simulink model "SYSTEM"  (R2026a)
settings: Solver=VariableStepAuto
model workspace (MAT data in the model file):
  CompAir_P : Simulink.ConnectionBus (value not decoded)
  CompAir_S : Simulink.Bus (value not decoded)
  Control_P : Simulink.ConnectionBus (value not decoded)
  Control_S : Simulink.Bus (value not decoded)
  CoolingFW_P : Simulink.ConnectionBus (value not decoded)
  CoolingFW_S : Simulink.Bus (value not decoded)
  FuelOil_P : Simulink.ConnectionBus (value not decoded)
  FuelOil_S : Simulink.Bus (value not decoded)
  Heat_P : Simulink.ConnectionBus (value not decoded)
  Heat_S : Simulink.Bus (value not decoded)
  LubeOil_P : Simulink.ConnectionBus (value not decoded)
  LubeOil_S : Simulink.Bus (value not decoded)
  Physical : Simulink.ConnectionBus (value not decoded)
  Power_P : Simulink.ConnectionBus (value not decoded)
  Power_S : Simulink.Bus (value not decoded)
  SaltWater_P : Simulink.ConnectionBus (value not decoded)
  SaltWater_S : Simulink.Bus (value not decoded)
  WasteGas_P : Simulink.ConnectionBus (value not decoded)
  WasteGas_S : Simulink.Bus (value not decoded)
  WasteOil_P : Simulink.ConnectionBus (value not decoded)
  WasteOil_S : Simulink.Bus (value not decoded)
  WasteSolid_P : Simulink.ConnectionBus (value not decoded)
  WasteSolid_S : Simulink.Bus (value not decoded)
  WasteWater_P : Simulink.ConnectionBus (value not decoded)
  WasteWater_S : Simulink.Bus (value not decoded)
undefined symbols (not defined in the file): FUEL
(part 3 of 5)

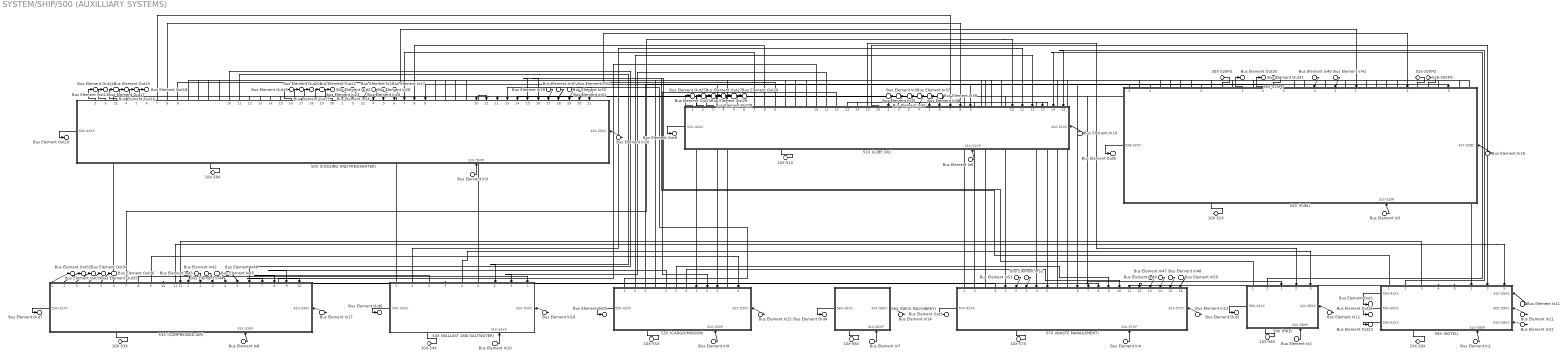
== system SYSTEM/SHIP/500 (AUXILLIARY SYSTEMS) ==
  Bus Element In23 : Inport  PortName=20X-50XCFW
  Bus Element In24 : Inport  Port=2  PortName=21X-50XCFW
  Bus Element In40 : Inport  Port=3  PortName=20X-52XFO
  Bus Element In42 : Inport  Port=4  PortName=20X-53XCA
  Bus Element In51 : Inport  Port=5  PortName=20X-57XWG
  Bus Element In25 : Inport  Port=6  PortName=30X-50XCFW
  Bus Element In28 : Inport  Port=7  PortName=42X-50XCFW
  Bus Element In43 : Inport  Port=8  PortName=21X-53XCA
  Bus Element In26 : Inport  Port=9  PortName=43X-50XCFW
  Bus Element In44 : Inport  Port=10  PortName=22X-53XCA
  Bus Element In27 : Inport  Port=11  PortName=44X-50XCFW
  Bus Element In29 : Inport  Port=12  PortName=60X-50XCFW
  Bus Element In38 : Inport  Port=13  PortName=30X-51XLO
  Bus Element In41 : Inport  Port=14  PortName=30X-52XFO
  Bus Element In45 : Inport  Port=15  PortName=30X-53XCA
  Bus Element In52 : Inport  Port=16  PortName=30X-57XWG
  Bus Element In46 : Inport  Port=17  PortName=40X-53XCA
  Bus Element In31 : Inport  Port=18  PortName=73X-50XCFW
  Bus Element In33 : Inport  Port=19  PortName=71X-50XCFW
  Bus Element In39 : Inport  Port=20  PortName=43X-51XLO
  Bus Element In32 : Inport  Port=21  PortName=72X-50XCFW
  Bus Element In30 : Inport  Port=22  PortName=61X-50XCFW
  Bus Element In47 : Inport  Port=23  PortName=60X-57XWW
  Bus Element In49 : Inport  Port=24  PortName=60X-57XWS
  Bus Element In34 : Inport  Port=25  PortName=20X-51XLO
  Bus Element In48 : Inport  Port=26  PortName=61X-57XWW
  Bus Element In50 : Inport  Port=27  PortName=61X-57XWS
  Bus Element In35 : Inport  Port=28  PortName=21X-51XLO
  Bus Element In36 : Inport  Port=29  PortName=22X-51XLO
  Bus Element In37 : Inport  Port=30  PortName=23X-51XLO
  Bus Element In20 : Inport  Port=31  PortName=42X-50XC
  Bus Element In19 : Inport  Port=32  PortName=42X-51XC
  Bus Element In18 : Inport  Port=33  PortName=42X-528C
  Bus Element In17 : Inport  Port=34  PortName=42X-53XC
  Bus Element In16 : Inport  Port=35  PortName=42X-54XC
  Bus Element In15 : Inport  Port=36  PortName=42X-55XC
  Bus Element In14 : Inport  Port=37  PortName=42X-56XC
  Bus Element In13 : Inport  Port=38  PortName=42X-57XC
  Bus Element In12 : Inport  Port=39  PortName=42X-58XC
  Bus Element In11 : Inport  Port=40  PortName=42X-59XC
  Bus Element In21 : Inport  Port=41  PortName=60X-59XC
  Bus Element In22 : Inport  Port=42  PortName=61X-59XC
  Bus Element In3 : Inport  Port=43  PortName=31X-50XP
  Bus Element In6 : Inport  Port=44  PortName=31X-51XP
  Bus Element In5 : Inport  Port=45  PortName=31X-529P
  Bus Element In8 : Inport  Port=46  PortName=31X-53XP
  Bus Element In10 : Inport  Port=47  PortName=31X-54XP
  Bus Element In9 : Inport  Port=48  PortName=31X-55XP
  Bus Element In7 : Inport  Port=49  PortName=31X-56XP
  Bus Element In4 : Inport  Port=50  PortName=31X-57XP
  Bus Element In2 : Inport  Port=51  PortName=31X-58XP
  Bus Element In1 : Inport  Port=52  PortName=31X-59XP
  50X (COOLING AND FRESHWATER) : Subsystem
      settings: PortSchema="{\"entries\":[{\"content\":{\"headerSize\":26,\"margin\":15,\"minimumSpacing\":25,\"sides\":[{\"content\":{\"connectorIds\":[\"Out1\"]},\"type\":\"ConnectorPlacement.EquallySpacedRectSide\",\"uuid\":\"c62bca68-e99b-4d4a-8c3b-c9a3c6520291\"},{\"content\":{\"connectorIds\":[\"In1\"],\"side\":\"RIGHT\"},\"type\":\"ConnectorPlacement.EquallySpacedRectSide\",\"uuid\":\"9f78cd75-5645-4950-8d66-9f0d33627f1f\"},{\"content\":{\"connectorIds\":[\"Out2\",\"Out3\",\"Out21\",\"Out4\",\"Out5\",\"Out6\",\"Out7\",\"Out8\",\"Out9\",\"LConn1\",\"LConn2\",\"LConn3\",\"LConn4\",\"Out10\",\"Out11\",\"Out12\",\"Out13\",\"Out14\",\"Out15\",\"Out16\",\"Out17\",\"Out18\",\"Out19\",\"Out20\",\"In2\",\"In3\",\"In22\",\"In4\",\"In5\",\"In6\",\"In7\",\"In8\",\"In9\",\"LConn5\",\"LConn6\",\"LConn7\",\"LConn8\",\"In10\",\"In12\",\"In11\",\"In13\",\"In14\",\"In15\",\"In16\",\"In17\",\"In18\",\"In19\",\"In20\",\"In21\"],\"side\":\"TOP\"},\"type\":\"ConnectorPlacement.EquallySpacedRectSide\",\"uuid\":\"f95077c9-4a6b-4bf1-8b13-59697d659817\"},{\"content\":{\"connectorIds\":[\"RConn1\",\"In23\"],\"side\":\"BOTTOM\"},\"type\":\"ConnectorPlacement.EquallySpacedRectSide\",\"uuid\":\"b0234a8b-87ef-4165-8ad1-aaed5018aad8\"}]},\"type\":\"ConnectorPlacement.EquallySpacedConnector\",\"uuid\":\"da1ef182-4ed3-4fb4-823f-e8eb0a5ecd15\"}],\"packageUris\":[\"http://schema.mathworks.com/mf0/Connector/R2020b\"],\"version\":\"1.0\"}"
  51X (LUBE OIL) : Subsystem
      settings: PortSchema="{\"entries\":[{\"content\":{\"headerSize\":26,\"margin\":15,\"minimumSpacing\":25,\"sides\":[{\"content\":{\"connectorIds\":[\"Out17\"]},\"type\":\"ConnectorPlacement.EquallySpacedRectSide\",\"uuid\":\"c62bca68-e99b-4d4a-8c3b-c9a3c6520291\"},{\"content\":{\"connectorIds\":[\"In16\"],\"side\":\"RIGHT\"},\"type\":\"ConnectorPlacement.EquallySpacedRectSide\",\"uuid\":\"9f78cd75-5645-4950-8d66-9f0d33627f1f\"},{\"content\":{\"connectorIds\":[\"Out1\",\"Out2\",\"Out3\",\"Out4\",\"Out5\",\"Out6\",\"Out7\",\"Out8\",\"Out9\",\"LConn1\",\"LConn2\",\"LConn3\",\"Out10\",\"Out11\",\"Out12\",\"Out13\",\"Out14\",\"Out15\",\"Out16\",\"In1\",\"In2\",\"In3\",\"In4\",\"In5\",\"In6\",\"In7\",\"In8\",\"In9\",\"LConn4\",\"LConn5\",\"LConn6\",\"In10\",\"In11\",\"In12\",\"In13\",\"In14\",\"In15\"],\"side\":\"TOP\"},\"type\":\"ConnectorPlacement.EquallySpacedRectSide\",\"uuid\":\"f95077c9-4a6b-4bf1-8b13-59697d659817\"},{\"content\":{\"connectorIds\":[\"RConn1\",\"In17\"],\"side\":\"BOTTOM\"},\"type\":\"ConnectorPlacement.EquallySpacedRectSide\",\"uuid\":\"d42e605c-5817-4d4d-affd-597e8c11adf0\"}]},\"type\":\"ConnectorPlacement.EquallySpacedConnector\",\"uuid\":\"da1ef182-4ed3-4fb4-823f-e8eb0a5ecd15\"}],\"packageUris\":[\"http://schema.mathworks.com/mf0/Connector/R2020b\"],\"version\":\"1.0\"}"
  52X (FUEL) : Subsystem  Variant=on  VariantControlMode=label  LabelModeActiveChoice=52X (FUEL)
      settings: PortSchema="{\"entries\":[{\"content\":{\"headerSize\":38,\"margin\":15,\"minimumSpacing\":25,\"sides\":[{\"content\":{\"connectorIds\":[\"Out7\"]},\"type\":\"ConnectorPlacement.EquallySpacedRectSide\",\"uuid\":\"c62bca68-e99b-4d4a-8c3b-c9a3c6520291\"},{\"content\":{\"connectorIds\":[\"In6\"],\"side\":\"RIGHT\"},\"type\":\"ConnectorPlacement.EquallySpacedRectSide\",\"uuid\":\"9f78cd75-5645-4950-8d66-9f0d33627f1f\"},{\"content\":{\"connectorIds\":[\"Out3\",\"LConn1\",\"Out4\",\"LConn9\",\"LConn2\",\"LConn10\",\"LConn3\",\"Out6\",\"LConn12\",\"LConn6\",\"LConn11\",\"Out1\",\"LConn4\",\"Out2\",\"LConn5\",\"Out5\",\"LConn8\",\"LConn7\",\"In4\",\"LConn13\",\"In2\",\"LConn14\",\"In1\",\"LConn15\",\"LConn16\",\"LConn17\",\"LConn18\",\"In3\",\"LConn19\",\"LConn20\",\"LConn21\",\"In5\",\"LConn22\",\"LConn23\"],\"side\":\"TOP\"},\"type\":\"ConnectorPlacement.EquallySpacedRectSide\",\"uuid\":\"f95077c9-4a6b-4bf1-8b13-59697d659817\"},{\"content\":{\"connectorIds\":[\"RConn1\",\"In7\"],\"side\":\"BOTTOM\"},\"type\":\"ConnectorPlacement.EquallySpacedRectSide\",\"uuid\":\"ebf76d24-9f66-4d93-ad0f-b873a6db50be\"}]},\"type\":\"ConnectorPlacement.EquallySpacedConnector\",\"uuid\":\"da1ef182-4ed3-4fb4-823f-e8eb0a5ecd15\"}],\"packageUris\":[\"http://schema.mathworks.com/mf0/Connector/R2020b\"],\"version\":\"1.0\"}"
  53X (COMPRESSED AIR) : Subsystem
      settings: PortSchema="{\"entries\":[{\"content\":{\"headerSize\":26,\"margin\":15,\"minimumSpacing\":25,\"sides\":[{\"content\":{\"connectorIds\":[\"Out12\"]},\"type\":\"ConnectorPlacement.EquallySpacedRectSide\",\"uuid\":\"c62bca68-e99b-4d4a-8c3b-c9a3c6520291\"},{\"content\":{\"connectorIds\":[\"In12\"],\"side\":\"RIGHT\"},\"type\":\"ConnectorPlacement.EquallySpacedRectSide\",\"uuid\":\"9f78cd75-5645-4950-8d66-9f0d33627f1f\"},{\"content\":{\"connectorIds\":[\"Out1\",\"Out2\",\"Out3\",\"Out4\",\"Out5\",\"Out6\",\"Out7\",\"Out8\",\"Out9\",\"Out10\",\"Out11\",\"In1\",\"In2\",\"In3\",\"In4\",\"In5\",\"In6\",\"In7\",\"In8\",\"In9\",\"In10\",\"In11\"],\"side\":\"TOP\"},\"type\":\"ConnectorPlacement.EquallySpacedRectSide\",\"uuid\":\"f95077c9-4a6b-4bf1-8b13-59697d659817\"},{\"content\":{\"connectorIds\":[\"RConn1\",\"In13\"],\"side\":\"BOTTOM\"},\"type\":\"ConnectorPlacement.EquallySpacedRectSide\",\"uuid\":\"5997a11e-7ecd-4610-be89-d40459c1eb53\"}]},\"type\":\"ConnectorPlacement.EquallySpacedConnector\",\"uuid\":\"da1ef182-4ed3-4fb4-823f-e8eb0a5ecd15\"}],\"packageUris\":[\"http://schema.mathworks.com/mf0/Connector/R2020b\"],\"version\":\"1.0\"}"
  54X (BALLAST AND SALTWATER) : Subsystem
      settings: PortSchema="{\"entries\":[{\"content\":{\"headerSize\":26,\"margin\":15,\"minimumSpacing\":25,\"sides\":[{\"content\":{\"connectorIds\":[\"Out7\"]},\"type\":\"ConnectorPlacement.EquallySpacedRectSide\",\"uuid\":\"c62bca68-e99b-4d4a-8c3b-c9a3c6520291\"},{\"content\":{\"connectorIds\":[\"In4\"],\"side\":\"RIGHT\"},\"type\":\"ConnectorPlacement.EquallySpacedRectSide\",\"uuid\":\"9f78cd75-5645-4950-8d66-9f0d33627f1f\"},{\"content\":{\"connectorIds\":[\"Out1\",\"Out2\",\"Out3\",\"Out5\",\"Out4\",\"Out6\",\"In2\",\"In3\",\"In1\"],\"side\":\"TOP\"},\"type\":\"ConnectorPlacement.EquallySpacedRectSide\",\"uuid\":\"f95077c9-4a6b-4bf1-8b13-59697d659817\"},{\"content\":{\"connectorIds\":[\"RConn1\",\"In5\"],\"side\":\"BOTTOM\"},\"type\":\"ConnectorPlacement.EquallySpacedRectSide\",\"uuid\":\"56267671-31b0-4414-99e2-68999b66eb0b\"}]},\"type\":\"ConnectorPlacement.EquallySpacedConnector\",\"uuid\":\"da1ef182-4ed3-4fb4-823f-e8eb0a5ecd15\"}],\"packageUris\":[\"http://schema.mathworks.com/mf0/Connector/R2020b\"],\"version\":\"1.0\"}"
  55X (CARGO/MISSION) : Subsystem
      settings: PortSchema="{\"entries\":[{\"content\":{\"headerSize\":26,\"margin\":15,\"minimumSpacing\":25,\"sides\":[{\"content\":{\"connectorIds\":[\"Out7\"]},\"type\":\"ConnectorPlacement.EquallySpacedRectSide\",\"uuid\":\"c62bca68-e99b-4d4a-8c3b-c9a3c6520291\"},{\"content\":{\"connectorIds\":[\"In5\"],\"side\":\"RIGHT\"},\"type\":\"ConnectorPlacement.EquallySpacedRectSide\",\"uuid\":\"9f78cd75-5645-4950-8d66-9f0d33627f1f\"},{\"content\":{\"connectorIds\":[\"Out1\",\"Out2\",\"Out3\",\"LConn1\",\"Out4\",\"Out5\",\"Out6\",\"In1\",\"In2\",\"In3\",\"LConn2\",\"In4\"],\"side\":\"TOP\"},\"type\":\"ConnectorPlacement.EquallySpacedRectSide\",\"uuid\":\"f95077c9-4a6b-4bf1-8b13-59697d659817\"},{\"content\":{\"connectorIds\":[\"RConn1\",\"In6\"],\"side\":\"BOTTOM\"},\"type\":\"ConnectorPlacement.EquallySpacedRectSide\",\"uuid\":\"0caecb8b-2871-432e-acc2-1a4670a43bd7\"}]},\"type\":\"ConnectorPlacement.EquallySpacedConnector\",\"uuid\":\"da1ef182-4ed3-4fb4-823f-e8eb0a5ecd15\"}],\"packageUris\":[\"http://schema.mathworks.com/mf0/Connector/R2020b\"],\"version\":\"1.0\"}"
  56X (DECK MACHINERY) : Subsystem
      settings: PortSchema="{\"entries\":[{\"content\":{\"headerSize\":26,\"margin\":15,\"minimumSpacing\":25,\"sides\":[{\"content\":{\"connectorIds\":[\"Out1\"]},\"type\":\"ConnectorPlacement.EquallySpacedRectSide\",\"uuid\":\"c62bca68-e99b-4d4a-8c3b-c9a3c6520291\"},{\"content\":{\"connectorIds\":[\"In1\"],\"side\":\"RIGHT\"},\"type\":\"ConnectorPlacement.EquallySpacedRectSide\",\"uuid\":\"9f78cd75-5645-4950-8d66-9f0d33627f1f\"},{\"content\":{\"side\":\"TOP\"},\"type\":\"ConnectorPlacement.EquallySpacedRectSide\",\"uuid\":\"f95077c9-4a6b-4bf1-8b13-59697d659817\"},{\"content\":{\"connectorIds\":[\"RConn1\",\"In2\"],\"side\":\"BOTTOM\"},\"type\":\"ConnectorPlacement.EquallySpacedRectSide\",\"uuid\":\"76c66af3-93a2-4131-95d6-01f8fd077363\"}]},\"type\":\"ConnectorPlacement.EquallySpacedConnector\",\"uuid\":\"da1ef182-4ed3-4fb4-823f-e8eb0a5ecd15\"}],\"packageUris\":[\"http://schema.mathworks.com/mf0/Connector/R2020b\"],\"version\":\"1.0\"}"
  57X (WASTE MANAGEMENT) : Subsystem
      settings: PortSchema="{\"entries\":[{\"content\":{\"headerSize\":26,\"margin\":15,\"minimumSpacing\":25,\"sides\":[{\"content\":{\"connectorIds\":[\"Out4\"]},\"type\":\"ConnectorPlacement.EquallySpacedRectSide\",\"uuid\":\"c62bca68-e99b-4d4a-8c3b-c9a3c6520291\"},{\"content\":{\"connectorIds\":[\"In17\"],\"side\":\"RIGHT\"},\"type\":\"ConnectorPlacement.EquallySpacedRectSide\",\"uuid\":\"9f78cd75-5645-4950-8d66-9f0d33627f1f\"},{\"content\":{\"connectorIds\":[\"Out1\",\"Out2\",\"LConn1\",\"Out3\",\"In1\",\"In2\",\"In3\",\"In4\",\"In5\",\"LConn2\",\"LConn3\",\"In6\",\"In7\",\"In8\",\"In9\",\"In10\",\"In11\",\"In12\",\"In13\",\"In14\",\"In15\",\"In16\"],\"side\":\"TOP\"},\"type\":\"ConnectorPlacement.EquallySpacedRectSide\",\"uuid\":\"f95077c9-4a6b-4bf1-8b13-59697d659817\"},{\"content\":{\"connectorIds\":[\"RConn1\",\"In18\"],\"side\":\"BOTTOM\"},\"type\":\"ConnectorPlacement.EquallySpacedRectSide\",\"uuid\":\"49855950-4e79-4387-81b7-3e6c63b80ca5\"}]},\"type\":\"ConnectorPlacement.EquallySpacedConnector\",\"uuid\":\"da1ef182-4ed3-4fb4-823f-e8eb0a5ecd15\"}],\"packageUris\":[\"http://schema.mathworks.com/mf0/Connector/R2020b\"],\"version\":\"1.0\"}"
  58X (FIRE) : Subsystem
      settings: PortSchema="{\"entries\":[{\"content\":{\"headerSize\":26,\"margin\":15,\"minimumSpacing\":25,\"sides\":[{\"content\":{\"connectorIds\":[\"Out3\"]},\"type\":\"ConnectorPlacement.EquallySpacedRectSide\",\"uuid\":\"c62bca68-e99b-4d4a-8c3b-c9a3c6520291\"},{\"content\":{\"connectorIds\":[\"In4\"],\"side\":\"RIGHT\"},\"type\":\"ConnectorPlacement.EquallySpacedRectSide\",\"uuid\":\"9f78cd75-5645-4950-8d66-9f0d33627f1f\"},{\"content\":{\"connectorIds\":[\"Out1\",\"Out2\",\"In1\",\"In2\",\"In3\"],\"side\":\"TOP\"},\"type\":\"ConnectorPlacement.EquallySpacedRectSide\",\"uuid\":\"f95077c9-4a6b-4bf1-8b13-59697d659817\"},{\"content\":{\"connectorIds\":[\"RConn1\",\"In5\"],\"side\":\"BOTTOM\"},\"type\":\"ConnectorPlacement.EquallySpacedRectSide\",\"uuid\":\"ddcbdc61-1e8a-4f23-9ee1-6302900fdae0\"}]},\"type\":\"ConnectorPlacement.EquallySpacedConnector\",\"uuid\":\"da1ef182-4ed3-4fb4-823f-e8eb0a5ecd15\"}],\"packageUris\":[\"http://schema.mathworks.com/mf0/Connector/R2020b\"],\"version\":\"1.0\"}"
  59X (HOTEL) : Subsystem
      settings: PortSchema="{\"entries\":[{\"content\":{\"headerSize\":26,\"margin\":15,\"minimumSpacing\":25,\"sides\":[{\"content\":{\"connectorIds\":[\"Out6\",\"Out7\",\"Out8\"]},\"type\":\"ConnectorPlacement.EquallySpacedRectSide\",\"uuid\":\"c62bca68-e99b-4d4a-8c3b-c9a3c6520291\"},{\"content\":{\"connectorIds\":[\"In4\",\"In5\",\"In6\"],\"side\":\"RIGHT\"},\"type\":\"ConnectorPlacement.EquallySpacedRectSide\",\"uuid\":\"9f78cd75-5645-4950-8d66-9f0d33627f1f\"},{\"content\":{\"connectorIds\":[\"Out1\",\"Out2\",\"Out3\",\"Out4\",\"Out5\",\"In1\",\"In2\",\"In3\"],\"side\":\"TOP\"},\"type\":\"ConnectorPlacement.EquallySpacedRectSide\",\"uuid\":\"f95077c9-4a6b-4bf1-8b13-59697d659817\"},{\"content\":{\"connectorIds\":[\"RConn1\",\"In7\"],\"side\":\"BOTTOM\"},\"type\":\"ConnectorPlacement.EquallySpacedRectSide\",\"uuid\":\"4cee84d2-0f5c-4d5e-8bc3-99a42f7ed665\"}]},\"type\":\"ConnectorPlacement.EquallySpacedConnector\",\"uuid\":\"da1ef182-4ed3-4fb4-823f-e8eb0a5ecd15\"}],\"packageUris\":[\"http://schema.mathworks.com/mf0/Connector/R2020b\"],\"version\":\"1.0\"}"
  525-20XFO : PMIOPort  Side=Left  ConnectionType=Bus: FuelOil_P
  526-30XFO : PMIOPort  Port=2  Side=Left  ConnectionType=Bus: FuelOil_P
  20X-525FO : PMIOPort  Port=3  Side=Left  ConnectionType=Bus: FuelOil_P
  30X-526FO : PMIOPort  Port=4  Side=Left  ConnectionType=Bus: FuelOil_P
  10X-50X : PMIOPort  Port=5  Side=Left  ConnectionType=Bus: Physical
  10X-51X : PMIOPort  Port=6  Side=Left  ConnectionType=Bus: Physical
  10X-52X : PMIOPort  Port=7  Side=Left  ConnectionType=Bus: Physical
  10X-53X : PMIOPort  Port=8  Side=Left  ConnectionType=Bus: Physical
  10X-54X : PMIOPort  Port=9  Side=Left  ConnectionType=Bus: Physical
  10X-55X : PMIOPort  Port=10  Side=Left  ConnectionType=Bus: Physical
  10X-56X : PMIOPort  Port=11  Side=Left  ConnectionType=Bus: Physical
  10X-57X : PMIOPort  Port=12  Side=Left  ConnectionType=Bus: Physical
  10X-58X : PMIOPort  Port=13  Side=Left  ConnectionType=Bus: Physical
  10X-59X : PMIOPort  Port=14  Side=Left  ConnectionType=Bus: Physical
  Bus Element Out14 : Outport  PortName=50X-20XCFW
  Bus Element Out13 : Outport  Port=2  PortName=50X-21XCFW
  Bus Element Out15 : Outport  Port=3  PortName=50X-30XCFW
  Bus Element Out17 : Outport  Port=4  PortName=50X-42XCFW
  Bus Element Out16 : Outport  Port=5  PortName=50X-43XCFW
  Bus Element Out18 : Outport  Port=6  PortName=50X-44XCFW
  Bus Element Out19 : Outport  Port=7  PortName=50X-60XCFW
  Bus Element Out20 : Outport  Port=8  PortName=50X-61XCFW
  Bus Element Out21 : Outport  Port=9  PortName=50X-71XCFW
  Bus Element Out22 : Outport  Port=10  PortName=50X-72XCFW
  Bus Element Out23 : Outport  Port=11  PortName=50X-73XCFW
  Bus Element Out24 : Outport  Port=12  PortName=51X-20XLO
  Bus Element Out25 : Outport  Port=13  PortName=51X-21XLO
  Bus Element Out26 : Outport  Port=14  PortName=51X-22XLO
  Bus Element Out27 : Outport  Port=15  PortName=51X-23XLO
  Bus Element Out28 : Outport  Port=16  PortName=51X-30XLO
  Bus Element Out29 : Outport  Port=17  PortName=51X-43XLO
  Bus Element Out30 : Outport  Port=18  PortName=52X-20XFO
  Bus Element Out31 : Outport  Port=19  PortName=52X-30XFO
  Bus Element Out32 : Outport  Port=20  PortName=53X-20XCA
  Bus Element Out33 : Outport  Port=21  PortName=53X-21XCA
  Bus Element Out34 : Outport  Port=22  PortName=53X-22XCA
  Bus Element Out35 : Outport  Port=23  PortName=53X-30XCA
  Bus Element Out36 : Outport  Port=24  PortName=53X-40XCA
  Bus Element Out10 : Outport  Port=25  PortName=50X-42XC
  Bus Element Out9 : Outport  Port=26  PortName=51X-42XC
  Bus Element Out8 : Outport  Port=27  PortName=528-42XC
  Bus Element Out7 : Outport  Port=28  PortName=53X-42XC
  Bus Element Out6 : Outport  Port=29  PortName=54X-42XC
  Bus Element Out5 : Outport  Port=30  PortName=55X-42XC
  Bus Element Out4 : Outport  Port=31  PortName=56X-42XC
  Bus Element Out3 : Outport  Port=32  PortName=57X-42XC
  Bus Element Out2 : Outport  Port=33  PortName=58X-42XC
  Bus Element Out1 : Outport  Port=34  PortName=59X-42XC
  Bus Element Out11 : Outport  Port=35  PortName=59X-60XC
  Bus Element Out12 : Outport  Port=36  PortName=59X-61XC
  wires:
  Bus Element In3/1 -> 50X (COOLING AND FRESHWATER)/23(31X-50XP)
  Bus Element In6/1 -> 51X (LUBE OIL)/17(31X-51XP)
  Bus Element In8/1 -> 53X (COMPRESSED AIR)/13(31X-53XP)
  Bus Element In10/1 -> 54X (BALLAST AND SALTWATER)/5(31X-54XP)
  Bus Element In9/1 -> 55X (CARGO/MISSION)/6(31X-55XP)
  Bus Element In7/1 -> 56X (DECK MACHINERY)/2(31X-56XP)
  Bus Element In4/1 -> 57X (WASTE MANAGEMENT)/18(31X-57XP)
  Bus Element In2/1 -> 58X (FIRE)/5(31X-58XP)
  Bus Element In1/1 -> 59X (HOTEL)/7(31X-59XP)
  Bus Element In20/1 -> 50X (COOLING AND FRESHWATER)/1(42X-50XC)
  Bus Element In19/1 -> 51X (LUBE OIL)/16(42X-51XC)
  Bus Element In17/1 -> 53X (COMPRESSED AIR)/12(42X-53XC)
  Bus Element In16/1 -> 54X (BALLAST AND SALTWATER)/4(42X-54XC)
  Bus Element In15/1 -> 55X (CARGO/MISSION)/5(42X-55XC)
  Bus Element In14/1 -> 56X (DECK MACHINERY)/1(42X-56XC)
  Bus Element In13/1 -> 57X (WASTE MANAGEMENT)/17(42X-57XC)
  Bus Element In12/1 -> 58X (FIRE)/4(42X-58XC)
  Bus Element In11/1 -> 59X (HOTEL)/4(42X-59XC)
  50X (COOLING AND FRESHWATER)/1(50X-42XC) -> Bus Element Out10/1
  51X (LUBE OIL)/17(51X-42XC) -> Bus Element Out9/1
  53X (COMPRESSED AIR)/12(53X-42XC) -> Bus Element Out7/1
  54X (BALLAST AND SALTWATER)/7(54X-42XC) -> Bus Element Out6/1
  55X (CARGO/MISSION)/7(55X-42XC) -> Bus Element Out5/1
  56X (DECK MACHINERY)/1(56X-42XC) -> Bus Element Out4/1
  57X (WASTE MANAGEMENT)/4(57X-42XC) -> Bus Element Out3/1
  58X (FIRE)/3(58X-42XC) -> Bus Element Out2/1
  59X (HOTEL)/6(59X-42XC) -> Bus Element Out1/1
  59X (HOTEL)/7(59X-60XC) -> Bus Element Out11/1
  59X (HOTEL)/8(59X-61XC) -> Bus Element Out12/1
  Bus Element In21/1 -> 59X (HOTEL)/5(60X-59XC)
  Bus Element In22/1 -> 59X (HOTEL)/6(61X-59XC)
  50X (COOLING AND FRESHWATER)/2(50X-20XCFW) -> Bus Element Out14/1
  50X (COOLING AND FRESHWATER)/3(50X-21XCFW) -> Bus Element Out13/1
  Bus Element In23/1 -> 50X (COOLING AND FRESHWATER)/2(20X-50XCFW)
  Bus Element In24/1 -> 50X (COOLING AND FRESHWATER)/3(21X-50XCFW)
  50X (COOLING AND FRESHWATER)/21(50X-30XCFW) -> Bus Element Out15/1
  Bus Element In25/1 -> 50X (COOLING AND FRESHWATER)/22(30X-50XCFW)
  50X (COOLING AND FRESHWATER)/5(50X-43XCFW) -> Bus Element Out16/1
  Bus Element In26/1 -> 50X (COOLING AND FRESHWATER)/5(43X-50XCFW)
  51X (LUBE OIL)/7(51X-50XCFW) -> 50X (COOLING AND FRESHWATER)/7(51X-50XCFW)
  50X (COOLING AND FRESHWATER)/7(50X-51XCFW) -> 51X (LUBE OIL)/7(50X-51XCFW)
  50X (COOLING AND FRESHWATER)/10(50X-53XCFW) -> 53X (COMPRESSED AIR)/6(50X-53XCFW)
  53X (COMPRESSED AIR)/6(53X-50XCFW) -> 50X (COOLING AND FRESHWATER)/10(53X-50XCFW)
  54X (BALLAST AND SALTWATER)/1(54X-50XSW) -> 50X (COOLING AND FRESHWATER)/11(54X-50XSW)
  54X (BALLAST AND SALTWATER)/4(54X-58XSW) -> 58X (FIRE)/3(54X-58XSW)
  54X (BALLAST AND SALTWATER)/5(54X-57XSW) -> 57X (WASTE MANAGEMENT)/8(54X-57XSW)
  54X (BALLAST AND SALTWATER)/6(54X-50XCFW) -> 50X (COOLING AND FRESHWATER)/12(54X-50XCFW)
  50X (COOLING AND FRESHWATER)/11(50X-54XCFW) -> 54X (BALLAST AND SALTWATER)/2(50X-54XCFW)
  50X (COOLING AND FRESHWATER)/12(50X-55XCFW) -> 55X (CARGO/MISSION)/1(50X-55XCFW)
  55X (CARGO/MISSION)/1(55X-50XCFW) -> 50X (COOLING AND FRESHWATER)/13(55X-50XCFW)
  57X (WASTE MANAGEMENT)/1(57X-50XCFW) -> 50X (COOLING AND FRESHWATER)/14(57X-50XCFW)
  50X (COOLING AND FRESHWATER)/13(50X-57XCFW) -> 57X (WASTE MANAGEMENT)/1(50X-57XCFW)
  58X (FIRE)/1(58X-50XCFW) -> 50X (COOLING AND FRESHWATER)/15(58X-50XCFW)
  59X (HOTEL)/1(59X-50XCFW) -> 50X (COOLING AND FRESHWATER)/16(59X-50XCFW)
  50X (COOLING AND FRESHWATER)/14(50X-58XCFW) -> 58X (FIRE)/1(50X-58XCFW)
  50X (COOLING AND FRESHWATER)/15(50X-59XCFW) -> 59X (HOTEL)/1(50X-59XCFW)
  50X (COOLING AND FRESHWATER)/4(50X-42XCFW) -> Bus Element Out17/1
  50X (COOLING AND FRESHWATER)/6(50X-44XCFW) -> Bus Element Out18/1
  Bus Element In28/1 -> 50X (COOLING AND FRESHWATER)/4(42X-50XCFW)
  Bus Element In27/1 -> 50X (COOLING AND FRESHWATER)/6(44X-50XCFW)
  50X (COOLING AND FRESHWATER)/16(50X-60XCFW) -> Bus Element Out19/1
  50X (COOLING AND FRESHWATER)/17(50X-61XCFW) -> Bus Element Out20/1
  50X (COOLING AND FRESHWATER)/18(50X-71XCFW) -> Bus Element Out21/1
  50X (COOLING AND FRESHWATER)/19(50X-72XCFW) -> Bus Element Out22/1
  50X (COOLING AND FRESHWATER)/20(50X-73XCFW) -> Bus Element Out23/1
  Bus Element In31/1 -> 50X (COOLING AND FRESHWATER)/21(73X-50XCFW)
  Bus Element In32/1 -> 50X (COOLING AND FRESHWATER)/20(72X-50XCFW)
  Bus Element In33/1 -> 50X (COOLING AND FRESHWATER)/19(71X-50XCFW)
  Bus Element In30/1 -> 50X (COOLING AND FRESHWATER)/18(61X-50XCFW)
  Bus Element In29/1 -> 50X (COOLING AND FRESHWATER)/17(60X-50XCFW)
  51X (LUBE OIL)/1(51X-20XLO) -> Bus Element Out24/1
  51X (LUBE OIL)/2(51X-21XLO) -> Bus Element Out25/1
  51X (LUBE OIL)/3(51X-22XLO) -> Bus Element Out26/1
  51X (LUBE OIL)/4(51X-23XLO) -> Bus Element Out27/1
  51X (LUBE OIL)/5(51X-30XLO) -> Bus Element Out28/1
  51X (LUBE OIL)/6(51X-43XLO) -> Bus Element Out29/1
  Bus Element In34/1 -> 51X (LUBE OIL)/1(20X-51XLO)
  Bus Element In35/1 -> 51X (LUBE OIL)/2(21X-51XLO)
  Bus Element In36/1 -> 51X (LUBE OIL)/3(22X-51XLO)
  Bus Element In37/1 -> 51X (LUBE OIL)/4(23X-51XLO)
  Bus Element In38/1 -> 51X (LUBE OIL)/5(30X-51XLO)
  Bus Element In39/1 -> 51X (LUBE OIL)/6(43X-51XLO)
  50X (COOLING AND FRESHWATER)/8(50X-51XLO) -> 51X (LUBE OIL)/8(50X-51XLO)
  51X (LUBE OIL)/8(51X-50XLO) -> 50X (COOLING AND FRESHWATER)/8(51X-50XLO)
  53X (COMPRESSED AIR)/7(53X-51XLO) -> 51X (LUBE OIL)/10(53X-51XLO)
  51X (LUBE OIL)/10(51X-53XLO) -> 53X (COMPRESSED AIR)/7(51X-53XLO)
  54X (BALLAST AND SALTWATER)/2(54X-51XLO) -> 51X (LUBE OIL)/11(54X-51XLO)
  51X (LUBE OIL)/11(51X-54XLO) -> 54X (BALLAST AND SALTWATER)/3(51X-54XLO)
  55X (CARGO/MISSION)/2(55X-51XLO) -> 51X (LUBE OIL)/12(55X-51XLO)
  51X (LUBE OIL)/12(51X-55XLO) -> 55X (CARGO/MISSION)/2(51X-55XLO)
  57X (WASTE MANAGEMENT)/2(57X-51XLO) -> 51X (LUBE OIL)/13(57X-51XLO)
  51X (LUBE OIL)/14(51X-57XLO) -> 57X (WASTE MANAGEMENT)/5(51X-57XLO)
  58X (FIRE)/2(58X-51XLO) -> 51X (LUBE OIL)/14(58X-51XLO)
  51X (LUBE OIL)/15(51X-58XLO) -> 58X (FIRE)/2(51X-58XLO)
  59X (HOTEL)/2(59X-51XLO) -> 51X (LUBE OIL)/15(59X-51XLO)
  51X (LUBE OIL)/16(51X-59XLO) -> 59X (HOTEL)/2(51X-59XLO)
  53X (COMPRESSED AIR)/1(53X-20XCA) -> Bus Element Out32/1
  53X (COMPRESSED AIR)/2(53X-21XCA) -> Bus Element Out33/1
  53X (COMPRESSED AIR)/3(53X-22XCA) -> Bus Element Out34/1
  53X (COMPRESSED AIR)/4(53X-30XCA) -> Bus Element Out35/1
  53X (COMPRESSED AIR)/5(53X-40XCA) -> Bus Element Out36/1
  Bus Element In42/1 -> 53X (COMPRESSED AIR)/1(20X-53XCA)
  Bus Element In43/1 -> 53X (COMPRESSED AIR)/2(21X-53XCA)
  Bus Element In44/1 -> 53X (COMPRESSED AIR)/3(22X-53XCA)
  Bus Element In45/1 -> 53X (COMPRESSED AIR)/4(30X-53XCA)
  Bus Element In46/1 -> 53X (COMPRESSED AIR)/5(40X-53XCA)
  54X (BALLAST AND SALTWATER)/3(54X-53XCA) -> 53X (COMPRESSED AIR)/8(54X-53XCA)
  55X (CARGO/MISSION)/4(55X-53XCA) -> 53X (COMPRESSED AIR)/9(55X-53XCA)
  57X (WASTE MANAGEMENT)/3(57X-53XCA) -> 53X (COMPRESSED AIR)/10(57X-53XCA)
  59X (HOTEL)/3(59X-53XCA) -> 53X (COMPRESSED AIR)/11(59X-53XCA)
  53X (COMPRESSED AIR)/8(53X-54XCA) -> 54X (BALLAST AND SALTWATER)/1(53X-54XCA)
  53X (COMPRESSED AIR)/9(53X-55XCA) -> 55X (CARGO/MISSION)/4(53X-55XCA)
  53X (COMPRESSED AIR)/10(53X-57XCA) -> 57X (WASTE MANAGEMENT)/7(53X-57XCA)
  53X (COMPRESSED AIR)/11(53X-59XCA) -> 59X (HOTEL)/3(53X-59XCA)
  Bus Element In47/1 -> 57X (WASTE MANAGEMENT)/13(60X-57XWW)
  Bus Element In48/1 -> 57X (WASTE MANAGEMENT)/15(61X-57XWW)
  59X (HOTEL)/4(59X-57XWW) -> 57X (WASTE MANAGEMENT)/11(59X-57XWW)
  55X (CARGO/MISSION)/5(55X-57XWW) -> 57X (WASTE MANAGEMENT)/9(55X-57XWW)
  51X (LUBE OIL)/13(51X-57XWO) -> 57X (WASTE MANAGEMENT)/4(51X-57XWO)
  Bus Element In49/1 -> 57X (WASTE MANAGEMENT)/14(60X-57XWS)
  Bus Element In50/1 -> 57X (WASTE MANAGEMENT)/16(61X-57XWS)
  55X (CARGO/MISSION)/6(55X-57XWS) -> 57X (WASTE MANAGEMENT)/10(55X-57XWS)
  59X (HOTEL)/5(59X-57XWS) -> 57X (WASTE MANAGEMENT)/12(59X-57XWS)
  Bus Element In51/1 -> 57X (WASTE MANAGEMENT)/2(20X-57XWG)
  Bus Element In52/1 -> 57X (WASTE MANAGEMENT)/3(30X-57XWG)
  50X (COOLING AND FRESHWATER)/9(50X-52XCFW) -> 52X (FUEL)/1(50X-52XCFW)
  Bus Element In41/1 -> 52X (FUEL)/2(30X-52XFO)
  51X (LUBE OIL)/9(51X-52XLO) -> 52X (FUEL)/3(51X-52XLO)
  Bus Element In40/1 -> 52X (FUEL)/4(20X-52XFO)
  55X (CARGO/MISSION)/3(55X-52XFO) -> 52X (FUEL)/5(55X-52XFO)
  Bus Element In18/1 -> 52X (FUEL)/6(42X-528C)
  Bus Element In5/1 -> 52X (FUEL)/7(31X-529P)
  52X (FUEL)/1(52X-20XFO) -> Bus Element Out30/1
  52X (FUEL)/2(52X-30XFO) -> Bus Element Out31/1
  52X (FUEL)/3(52X-50XCFW) -> 50X (COOLING AND FRESHWATER)/9(52X-50XCFW)
  52X (FUEL)/4(52X-51XLO) -> 51X (LUBE OIL)/9(52X-51XLO)
  52X (FUEL)/5(52X-55XFO) -> 55X (CARGO/MISSION)/3(52X-55XFO)
  52X (FUEL)/6(52X-57XWO) -> 57X (WASTE MANAGEMENT)/6(52X-57XWO)
  52X (FUEL)/7(528-42XC) -> Bus Element Out8/1
  connections:
  50X (COOLING AND FRESHWATER)/RConn1 -- 10X-50X/RConn1
  51X (LUBE OIL)/RConn1 -- 10X-51X/RConn1
  53X (COMPRESSED AIR)/RConn1 -- 10X-53X/RConn1
  54X (BALLAST AND SALTWATER)/RConn1 -- 10X-54X/RConn1
  55X (CARGO/MISSION)/RConn1 -- 10X-55X/RConn1
  56X (DECK MACHINERY)/RConn1 -- 10X-56X/RConn1
  57X (WASTE MANAGEMENT)/RConn1 -- 10X-57X/RConn1
  58X (FIRE)/RConn1 -- 10X-58X/RConn1
  59X (HOTEL)/RConn1 -- 10X-59X/RConn1
  52X (FUEL)/LConn11 -- 50X (COOLING AND FRESHWATER)/LConn5
  52X (FUEL)/LConn17 -- 50X (COOLING AND FRESHWATER)/LConn6
  52X (FUEL)/LConn18 -- 57X (WASTE MANAGEMENT)/LConn2
  52X (FUEL)/LConn19 -- 525-20XFO/RConn1
  52X (FUEL)/LConn20 -- 526-30XFO/RConn1
  52X (FUEL)/LConn21 -- 50X (COOLING AND FRESHWATER)/LConn7
  52X (FUEL)/LConn22 -- 50X (COOLING AND FRESHWATER)/LConn8
  52X (FUEL)/LConn23 -- 55X (CARGO/MISSION)/LConn2
  52X (FUEL)/LConn1 -- 51X (LUBE OIL)/LConn4
  52X (FUEL)/LConn2 -- 51X (LUBE OIL)/LConn5
  52X (FUEL)/LConn3 -- 51X (LUBE OIL)/LConn6
  52X (FUEL)/LConn4 -- 57X (WASTE MANAGEMENT)/LConn3
  52X (FUEL)/LConn5 -- 20X-525FO/RConn1
  52X (FUEL)/LConn6 -- 30X-526FO/RConn1
  52X (FUEL)/LConn7 -- 50X (COOLING AND FRESHWATER)/LConn1
  52X (FUEL)/LConn8 -- 50X (COOLING AND FRESHWATER)/LConn2
  52X (FUEL)/LConn9 -- 50X (COOLING AND FRESHWATER)/LConn3
  52X (FUEL)/LConn10 -- 50X (COOLING AND FRESHWATER)/LConn4
  52X (FUEL)/LConn12 -- 51X (LUBE OIL)/LConn1
  52X (FUEL)/LConn13 -- 51X (LUBE OIL)/LConn2
  52X (FUEL)/LConn14 -- 51X (LUBE OIL)/LConn3
  52X (FUEL)/LConn15 -- 55X (CARGO/MISSION)/LConn1
  52X (FUEL)/LConn16 -- 57X (WASTE MANAGEMENT)/LConn1
  52X (FUEL)/RConn1 -- 10X-52X/RConn1

== system SYSTEM/SHIP/600 (OUTFITTING) ==
  Bus Element In5 : Inport  PortName=50X-60XCFW
  Bus Element In6 : Inport  Port=2  PortName=50X-61XCFW
  Bus Element In4 : Inport  Port=3  PortName=59X-60XC
  Bus Element In3 : Inport  Port=4  PortName=59X-61XC
  Bus Element In1 : Inport  Port=5  PortName=31X-60XP
  Bus Element In2 : Inport  Port=6  PortName=31X-61XP
  60X (ACCOMODATION) : Subsystem
      settings: PortSchema="{\"entries\":[{\"content\":{\"headerSize\":26,\"margin\":15,\"minimumSpacing\":25,\"sides\":[{\"content\":{\"connectorIds\":[\"Out4\"]},\"type\":\"ConnectorPlacement.EquallySpacedRectSide\",\"uuid\":\"c62bca68-e99b-4d4a-8c3b-c9a3c6520291\"},{\"content\":{\"connectorIds\":[\"In2\"],\"side\":\"RIGHT\"},\"type\":\"ConnectorPlacement.EquallySpacedRectSide\",\"uuid\":\"9f78cd75-5645-4950-8d66-9f0d33627f1f\"},{\"content\":{\"connectorIds\":[\"Out1\",\"Out2\",\"Out3\",\"In1\"],\"side\":\"TOP\"},\"type\":\"ConnectorPlacement.EquallySpacedRectSide\",\"uuid\":\"f95077c9-4a6b-4bf1-8b13-59697d659817\"},{\"content\":{\"connectorIds\":[\"RConn1\",\"In3\"],\"side\":\"BOTTOM\"},\"type\":\"ConnectorPlacement.EquallySpacedRectSide\",\"uuid\":\"173b5817-d8cb-4853-b360-af39f3476a89\"}]},\"type\":\"ConnectorPlacement.EquallySpacedConnector\",\"uuid\":\"da1ef182-4ed3-4fb4-823f-e8eb0a5ecd15\"}],\"packageUris\":[\"http://schema.mathworks.com/mf0/Connector/R2020b\"],\"version\":\"1.0\"}"
  61X (SHOPS) : Subsystem
      settings: PortSchema="{\"entries\":[{\"content\":{\"headerSize\":26,\"margin\":15,\"minimumSpacing\":25,\"sides\":[{\"content\":{\"connectorIds\":[\"Out4\"]},\"type\":\"ConnectorPlacement.EquallySpacedRectSide\",\"uuid\":\"c62bca68-e99b-4d4a-8c3b-c9a3c6520291\"},{\"content\":{\"connectorIds\":[\"In2\"],\"side\":\"RIGHT\"},\"type\":\"ConnectorPlacement.EquallySpacedRectSide\",\"uuid\":\"9f78cd75-5645-4950-8d66-9f0d33627f1f\"},{\"content\":{\"connectorIds\":[\"Out1\",\"Out2\",\"Out3\",\"In1\"],\"side\":\"TOP\"},\"type\":\"ConnectorPlacement.EquallySpacedRectSide\",\"uuid\":\"f95077c9-4a6b-4bf1-8b13-59697d659817\"},{\"content\":{\"connectorIds\":[\"RConn1\",\"In3\"],\"side\":\"BOTTOM\"},\"type\":\"ConnectorPlacement.EquallySpacedRectSide\",\"uuid\":\"8e5207f0-8fd0-4632-9b54-d721f4677083\"}]},\"type\":\"ConnectorPlacement.EquallySpacedConnector\",\"uuid\":\"da1ef182-4ed3-4fb4-823f-e8eb0a5ecd15\"}],\"packageUris\":[\"http://schema.mathworks.com/mf0/Connector/R2020b\"],\"version\":\"1.0\"}"
  62X (LSA) : Subsystem
      settings: PortSchema="{\"entries\":[{\"content\":{\"headerSize\":26,\"margin\":15,\"minimumSpacing\":25,\"sides\":[{\"content\":{},\"type\":\"ConnectorPlacement.EquallySpacedRectSide\",\"uuid\":\"c62bca68-e99b-4d4a-8c3b-c9a3c6520291\"},{\"content\":{\"side\":\"RIGHT\"},\"type\":\"ConnectorPlacement.EquallySpacedRectSide\",\"uuid\":\"9f78cd75-5645-4950-8d66-9f0d33627f1f\"},{\"content\":{\"side\":\"TOP\"},\"type\":\"ConnectorPlacement.EquallySpacedRectSide\",\"uuid\":\"f95077c9-4a6b-4bf1-8b13-59697d659817\"},{\"content\":{\"connectorIds\":[\"RConn1\"],\"side\":\"BOTTOM\"},\"type\":\"ConnectorPlacement.EquallySpacedRectSide\",\"uuid\":\"1eb5152a-d644-438e-ab5b-d56f1840f95d\"}]},\"type\":\"ConnectorPlacement.EquallySpacedConnector\",\"uuid\":\"da1ef182-4ed3-4fb4-823f-e8eb0a5ecd15\"}],\"packageUris\":[\"http://schema.mathworks.com/mf0/Connector/R2020b\"],\"version\":\"1.0\"}"
  10X-60X : PMIOPort  Side=Left  ConnectionType=Bus: Physical
  10X-61X : PMIOPort  Port=2  Side=Left  ConnectionType=Bus: Physical
  10X-62X : PMIOPort  Port=3  Side=Left  ConnectionType=Bus: Physical
  Bus Element Out3 : Outport  PortName=60X-50XCFW
  Bus Element Out5 : Outport  Port=2  PortName=60X-57XWW
  Bus Element Out7 : Outport  Port=3  PortName=60X-57XWS
  Bus Element Out4 : Outport  Port=4  PortName=61X-50XCFW
  Bus Element Out6 : Outport  Port=5  PortName=61X-57XWW
  Bus Element Out8 : Outport  Port=6  PortName=61X-57XWS
  Bus Element Out1 : Outport  Port=7  PortName=60X-59XC
  Bus Element Out2 : Outport  Port=8  PortName=61X-59XC
  wires:
  Bus Element In1/1 -> 60X (ACCOMODATION)/3(31X-60XP)
  Bus Element In2/1 -> 61X (SHOPS)/3(31X-61XP)
  Bus Element In4/1 -> 60X (ACCOMODATION)/2(59X-60XC)
  Bus Element In3/1 -> 61X (SHOPS)/2(59X-61XC)
  61X (SHOPS)/4(61X-59XC) -> Bus Element Out2/1
  60X (ACCOMODATION)/4(60X-59XC) -> Bus Element Out1/1
  60X (ACCOMODATION)/1(60X-50XCFW) -> Bus Element Out3/1
  61X (SHOPS)/1(61X-50XCFW) -> Bus Element Out4/1
  Bus Element In5/1 -> 60X (ACCOMODATION)/1(50X-60XCFW)
  Bus Element In6/1 -> 61X (SHOPS)/1(50X-61XCFW)
  60X (ACCOMODATION)/2(60X-57XWW) -> Bus Element Out5/1
  61X (SHOPS)/2(61X-57XWW) -> Bus Element Out6/1
  60X (ACCOMODATION)/3(60X-57XWS) -> Bus Element Out7/1
  61X (SHOPS)/3(61X-57XWS) -> Bus Element Out8/1
  connections:
  60X (ACCOMODATION)/RConn1 -- 10X-60X/RConn1
  61X (SHOPS)/RConn1 -- 10X-61X/RConn1
  62X (LSA)/RConn1 -- 10X-62X/RConn1

== system SYSTEM/SHIP/700 (WEAPONS) ==
  Bus Element In11 : Inport  PortName=50X-71XCFW
  Bus Element In12 : Inport  Port=2  PortName=50X-72XCFW
  Bus Element In13 : Inport  Port=3  PortName=50X-73XCFW
  Bus Element In6 : Inport  Port=4  PortName=42X-70XC
  Bus Element In7 : Inport  Port=5  PortName=42X-71XC
  Bus Element In8 : Inport  Port=6  PortName=42X-72XC
  Bus Element In9 : Inport  Port=7  PortName=42X-73XC
  Bus Element In10 : Inport  Port=8  PortName=42X-74XC
  Bus Element In1 : Inport  Port=9  PortName=31X-70XP
  Bus Element In3 : Inport  Port=10  PortName=31X-71XP
  Bus Element In4 : Inport  Port=11  PortName=31X-72XP
  Bus Element In5 : Inport  Port=12  PortName=31X-73XP
  Bus Element In2 : Inport  Port=13  PortName=31X-74XP
  70X (ASW) : Subsystem
      settings: PortSchema="{\"entries\":[{\"content\":{\"headerSize\":26,\"margin\":15,\"minimumSpacing\":25,\"sides\":[{\"content\":{\"connectorIds\":[\"Out1\"]},\"type\":\"ConnectorPlacement.EquallySpacedRectSide\",\"uuid\":\"c62bca68-e99b-4d4a-8c3b-c9a3c6520291\"},{\"content\":{\"connectorIds\":[\"In1\"],\"side\":\"RIGHT\"},\"type\":\"ConnectorPlacement.EquallySpacedRectSide\",\"uuid\":\"9f78cd75-5645-4950-8d66-9f0d33627f1f\"},{\"content\":{\"side\":\"TOP\"},\"type\":\"ConnectorPlacement.EquallySpacedRectSide\",\"uuid\":\"f95077c9-4a6b-4bf1-8b13-59697d659817\"},{\"content\":{\"connectorIds\":[\"RConn1\",\"In2\"],\"side\":\"BOTTOM\"},\"type\":\"ConnectorPlacement.EquallySpacedRectSide\",\"uuid\":\"ca7b3728-805b-4b40-a070-e0da1c1f7e0e\"}]},\"type\":\"ConnectorPlacement.EquallySpacedConnector\",\"uuid\":\"da1ef182-4ed3-4fb4-823f-e8eb0a5ecd15\"}],\"packageUris\":[\"http://schema.mathworks.com/mf0/Connector/R2020b\"],\"version\":\"1.0\"}"
  71X (SS) : Subsystem
      settings: PortSchema="{\"entries\":[{\"content\":{\"headerSize\":26,\"margin\":15,\"minimumSpacing\":25,\"sides\":[{\"content\":{\"connectorIds\":[\"Out2\"]},\"type\":\"ConnectorPlacement.EquallySpacedRectSide\",\"uuid\":\"c62bca68-e99b-4d4a-8c3b-c9a3c6520291\"},{\"content\":{\"connectorIds\":[\"In2\"],\"side\":\"RIGHT\"},\"type\":\"ConnectorPlacement.EquallySpacedRectSide\",\"uuid\":\"9f78cd75-5645-4950-8d66-9f0d33627f1f\"},{\"content\":{\"connectorIds\":[\"Out1\",\"In1\"],\"side\":\"TOP\"},\"type\":\"ConnectorPlacement.EquallySpacedRectSide\",\"uuid\":\"f95077c9-4a6b-4bf1-8b13-59697d659817\"},{\"content\":{\"connectorIds\":[\"RConn1\",\"In3\"],\"side\":\"BOTTOM\"},\"type\":\"ConnectorPlacement.EquallySpacedRectSide\",\"uuid\":\"329e0e2e-836e-4776-898e-98e4e50379fd\"}]},\"type\":\"ConnectorPlacement.EquallySpacedConnector\",\"uuid\":\"da1ef182-4ed3-4fb4-823f-e8eb0a5ecd15\"}],\"packageUris\":[\"http://schema.mathworks.com/mf0/Connector/R2020b\"],\"version\":\"1.0\"}"
  72X (SA) : Subsystem
      settings: PortSchema="{\"entries\":[{\"content\":{\"headerSize\":26,\"margin\":15,\"minimumSpacing\":25,\"sides\":[{\"content\":{\"connectorIds\":[\"Out2\"]},\"type\":\"ConnectorPlacement.EquallySpacedRectSide\",\"uuid\":\"c62bca68-e99b-4d4a-8c3b-c9a3c6520291\"},{\"content\":{\"connectorIds\":[\"In2\"],\"side\":\"RIGHT\"},\"type\":\"ConnectorPlacement.EquallySpacedRectSide\",\"uuid\":\"9f78cd75-5645-4950-8d66-9f0d33627f1f\"},{\"content\":{\"connectorIds\":[\"Out1\",\"In1\"],\"side\":\"TOP\"},\"type\":\"ConnectorPlacement.EquallySpacedRectSide\",\"uuid\":\"f95077c9-4a6b-4bf1-8b13-59697d659817\"},{\"content\":{\"connectorIds\":[\"RConn1\",\"In3\"],\"side\":\"BOTTOM\"},\"type\":\"ConnectorPlacement.EquallySpacedRectSide\",\"uuid\":\"c2e6e1dd-22b0-4490-bd6f-e92fdab27d04\"}]},\"type\":\"ConnectorPlacement.EquallySpacedConnector\",\"uuid\":\"da1ef182-4ed3-4fb4-823f-e8eb0a5ecd15\"}],\"packageUris\":[\"http://schema.mathworks.com/mf0/Connector/R2020b\"],\"version\":\"1.0\"}"
  73X (EW) : Subsystem
      settings: PortSchema="{\"entries\":[{\"content\":{\"headerSize\":26,\"margin\":15,\"minimumSpacing\":25,\"sides\":[{\"content\":{\"connectorIds\":[\"Out2\"]},\"type\":\"ConnectorPlacement.EquallySpacedRectSide\",\"uuid\":\"c62bca68-e99b-4d4a-8c3b-c9a3c6520291\"},{\"content\":{\"connectorIds\":[\"In2\"],\"side\":\"RIGHT\"},\"type\":\"ConnectorPlacement.EquallySpacedRectSide\",\"uuid\":\"9f78cd75-5645-4950-8d66-9f0d33627f1f\"},{\"content\":{\"connectorIds\":[\"Out1\",\"In1\"],\"side\":\"TOP\"},\"type\":\"ConnectorPlacement.EquallySpacedRectSide\",\"uuid\":\"f95077c9-4a6b-4bf1-8b13-59697d659817\"},{\"content\":{\"connectorIds\":[\"RConn1\",\"In3\"],\"side\":\"BOTTOM\"},\"type\":\"ConnectorPlacement.EquallySpacedRectSide\",\"uuid\":\"795392ee-6c21-43e3-b9cf-289e3e85a737\"}]},\"type\":\"ConnectorPlacement.EquallySpacedConnector\",\"uuid\":\"da1ef182-4ed3-4fb4-823f-e8eb0a5ecd15\"}],\"packageUris\":[\"http://schema.mathworks.com/mf0/Connector/R2020b\"],\"version\":\"1.0\"}"
  74X (COUNTERMEASURES) : Subsystem
      settings: PortSchema="{\"entries\":[{\"content\":{\"headerSize\":26,\"margin\":15,\"minimumSpacing\":25,\"sides\":[{\"content\":{\"connectorIds\":[\"Out1\"]},\"type\":\"ConnectorPlacement.EquallySpacedRectSide\",\"uuid\":\"c62bca68-e99b-4d4a-8c3b-c9a3c6520291\"},{\"content\":{\"connectorIds\":[\"In1\"],\"side\":\"RIGHT\"},\"type\":\"ConnectorPlacement.EquallySpacedRectSide\",\"uuid\":\"9f78cd75-5645-4950-8d66-9f0d33627f1f\"},{\"content\":{\"side\":\"TOP\"},\"type\":\"ConnectorPlacement.EquallySpacedRectSide\",\"uuid\":\"f95077c9-4a6b-4bf1-8b13-59697d659817\"},{\"content\":{\"connectorIds\":[\"RConn1\",\"In2\"],\"side\":\"BOTTOM\"},\"type\":\"ConnectorPlacement.EquallySpacedRectSide\",\"uuid\":\"c18ac205-e4c9-4f12-a538-f65cf59c4805\"}]},\"type\":\"ConnectorPlacement.EquallySpacedConnector\",\"uuid\":\"da1ef182-4ed3-4fb4-823f-e8eb0a5ecd15\"}],\"packageUris\":[\"http://schema.mathworks.com/mf0/Connector/R2020b\"],\"version\":\"1.0\"}"
  10X-70X : PMIOPort  Side=Left  ConnectionType=Bus: Physical
  10X-71X : PMIOPort  Port=2  Side=Left  ConnectionType=Bus: Physical
  10X-72X : PMIOPort  Port=3  Side=Left  ConnectionType=Bus: Physical
  10X-73X : PMIOPort  Port=4  Side=Left  ConnectionType=Bus: Physical
  10X-74X : PMIOPort  Port=5  Side=Left  ConnectionType=Bus: Physical
  Bus Element Out6 : Outport  PortName=71X-50XCFW
  Bus Element Out7 : Outport  Port=2  PortName=72X-50XCFW
  Bus Element Out8 : Outport  Port=3  PortName=73X-50XCFW
  Bus Element Out1 : Outport  Port=4  PortName=70X-42XC
  Bus Element Out2 : Outport  Port=5  PortName=71X-42XC
  Bus Element Out3 : Outport  Port=6  PortName=72X-42XC
  Bus Element Out4 : Outport  Port=7  PortName=73X-42XC
  Bus Element Out5 : Outport  Port=8  PortName=74X-42XC
  wires:
  Bus Element In1/1 -> 70X (ASW)/2(31X-70XP)
  Bus Element In3/1 -> 71X (SS)/3(31X-71XP)
  Bus Element In4/1 -> 72X (SA)/3(31X-72XP)
  Bus Element In5/1 -> 73X (EW)/3(31X-73XP)
  Bus Element In2/1 -> 74X (COUNTERMEASURES)/2(31X-74XP)
  Bus Element In6/1 -> 70X (ASW)/1(42X-70XC)
  Bus Element In7/1 -> 71X (SS)/2(42X-71XC)
  Bus Element In8/1 -> 72X (SA)/2(42X-72XC)
  Bus Element In9/1 -> 73X (EW)/2(42X-73XC)
  Bus Element In10/1 -> 74X (COUNTERMEASURES)/1(42X-74XC)
  70X (ASW)/1(70X-42XC) -> Bus Element Out1/1
  71X (SS)/2(71X-42XC) -> Bus Element Out2/1
  72X (SA)/2(72X-42XC) -> Bus Element Out3/1
  73X (EW)/2(73X-42XC) -> Bus Element Out4/1
  74X (COUNTERMEASURES)/1(74X-42XC) -> Bus Element Out5/1
  71X (SS)/1(71X-50XCFW) -> Bus Element Out6/1
  72X (SA)/1(72X-50XCFW) -> Bus Element Out7/1
  73X (EW)/1(73X-50XCFW) -> Bus Element Out8/1
  Bus Element In11/1 -> 71X (SS)/1(50X-71XCFW)
  Bus Element In12/1 -> 72X (SA)/1(50X-72XCFW)
  Bus Element In13/1 -> 73X (EW)/1(50X-73XCFW)
  connections:
  70X (ASW)/RConn1 -- 10X-70X/RConn1
  71X (SS)/RConn1 -- 10X-71X/RConn1
  72X (SA)/RConn1 -- 10X-72X/RConn1
  73X (EW)/RConn1 -- 10X-73X/RConn1
  74X (COUNTERMEASURES)/RConn1 -- 10X-74X/RConn1

== system SYSTEM/SHIP/100 (HULL)/10X (PLATE) ==
  W12X : PMIOPort  Side=Right  ConnectionType=Bus: Physical
  W11X : PMIOPort  Port=2  Side=Right  ConnectionType=Bus: Physical
  W20X : PMIOPort  Port=3  Side=Right  ConnectionType=Bus: Physical
  W21X : PMIOPort  Port=4  Side=Right  ConnectionType=Bus: Physical
  W22X : PMIOPort  Port=5  Side=Right  ConnectionType=Bus: Physical
  W23X : PMIOPort  Port=6  Side=Right  ConnectionType=Bus: Physical
  W30X : PMIOPort  Port=7  Side=Right  ConnectionType=Bus: Physical
  W31X : PMIOPort  Port=8  Side=Right  ConnectionType=Bus: Physical
  W32X : PMIOPort  Port=9  Side=Right  ConnectionType=Bus: Physical
  W33X : PMIOPort  Port=10  Side=Right  ConnectionType=Bus: Physical
  W40X : PMIOPort  Port=11  Side=Right  ConnectionType=Bus: Physical
  W41X : PMIOPort  Port=12  Side=Right  ConnectionType=Bus: Physical
  W42X : PMIOPort  Port=13  Side=Right  ConnectionType=Bus: Physical
  W43X : PMIOPort  Port=14  Side=Right  ConnectionType=Bus: Physical
  W44X : PMIOPort  Port=15  Side=Right  ConnectionType=Bus: Physical
  W45X : PMIOPort  Port=16  Side=Right  ConnectionType=Bus: Physical
  W50X : PMIOPort  Port=17  Side=Right  ConnectionType=Bus: Physical
  W51X : PMIOPort  Port=18  Side=Right  ConnectionType=Bus: Physical
  W52X : PMIOPort  Port=19  Side=Right  ConnectionType=Bus: Physical
  W53X : PMIOPort  Port=20  Side=Right  ConnectionType=Bus: Physical
  W54X : PMIOPort  Port=21  Side=Right  ConnectionType=Bus: Physical
  W55X : PMIOPort  Port=22  Side=Right  ConnectionType=Bus: Physical
  W56X : PMIOPort  Port=23  Side=Right  ConnectionType=Bus: Physical
  W57X : PMIOPort  Port=24  Side=Right  ConnectionType=Bus: Physical
  W58X : PMIOPort  Port=25  Side=Right  ConnectionType=Bus: Physical
  W59X : PMIOPort  Port=26  Side=Right  ConnectionType=Bus: Physical
  W60X : PMIOPort  Port=27  Side=Right  ConnectionType=Bus: Physical
  W61X : PMIOPort  Port=28  Side=Right  ConnectionType=Bus: Physical
  W62X : PMIOPort  Port=29  Side=Right  ConnectionType=Bus: Physical
  W70X : PMIOPort  Port=30  Side=Right  ConnectionType=Bus: Physical
  W71X : PMIOPort  Port=31  Side=Right  ConnectionType=Bus: Physical
  W72X : PMIOPort  Port=32  Side=Right  ConnectionType=Bus: Physical
  W73X : PMIOPort  Port=33  Side=Right  ConnectionType=Bus: Physical
  W74X : PMIOPort  Port=34  Side=Right  ConnectionType=Bus: Physical

== system SYSTEM/SHIP/100 (HULL)/11X (FRAMING) ==
  W10X : PMIOPort  Side=Left  ConnectionType=Bus: Physical
  W12X : PMIOPort  Port=2  Side=Right  ConnectionType=Bus: Physical

== system SYSTEM/SHIP/100 (HULL)/12X (STIFFENERS) ==
  W10X : PMIOPort  Side=Left  ConnectionType=Bus: Physical
  W11X : PMIOPort  Port=2  Side=Left  ConnectionType=Bus: Physical

== system SYSTEM/SHIP/200 (PROPULSION)/20X (MAIN ENGINE) ==
  42X-20XC : Inport  OutDataTypeStr=Bus: Control_S
  51X-20XLO : Inport  Port=2  OutDataTypeStr=Bus: LubeOil_S
  52X-20XFO : Inport  Port=3  OutDataTypeStr=Bus: FuelOil_S
  53X-20XCA : Inport  Port=4  OutDataTypeStr=Bus: CompAir_S
  50X-20XCFW : Inport  Port=5  OutDataTypeStr=Bus: CoolingFW_S
  20X ABSENT : Subsystem  VariantControl=20X ABSENT
      settings: PortSchema="{\"entries\":[{\"content\":{\"headerSize\":26,\"margin\":15,\"minimumSpacing\":25,\"sides\":[{\"content\":{},\"type\":\"ConnectorPlacement.EquallySpacedRectSide\",\"uuid\":\"c62bca68-e99b-4d4a-8c3b-c9a3c6520291\"},{\"content\":{\"side\":\"RIGHT\"},\"type\":\"ConnectorPlacement.EquallySpacedRectSide\",\"uuid\":\"9f78cd75-5645-4950-8d66-9f0d33627f1f\"},{\"content\":{\"side\":\"TOP\"},\"type\":\"ConnectorPlacement.EquallySpacedRectSide\",\"uuid\":\"f95077c9-4a6b-4bf1-8b13-59697d659817\"},{\"content\":{\"side\":\"BOTTOM\"},\"type\":\"ConnectorPlacement.EquallySpacedRectSide\",\"uuid\":\"0eafd906-a166-4c55-8e00-9a076c1e2d64\"}]},\"type\":\"ConnectorPlacement.EquallySpacedConnector\",\"uuid\":\"da1ef182-4ed3-4fb4-823f-e8eb0a5ecd15\"}],\"packageUris\":[\"http://schema.mathworks.com/mf0/Connector/R2020b\"],\"version\":\"1.0\"}"
  20X DIESEL ENGINE : Subsystem  VariantControl=20X DIESEL ENGINE
      settings: PortSchema="{\"entries\":[{\"content\":{\"headerSize\":26,\"margin\":15,\"minimumSpacing\":25,\"sides\":[{\"content\":{\"connectorIds\":[\"Out1\"]},\"type\":\"ConnectorPlacement.EquallySpacedRectSide\",\"uuid\":\"c62bca68-e99b-4d4a-8c3b-c9a3c6520291\"},{\"content\":{\"connectorIds\":[\"LConn3\",\"In1\"],\"side\":\"RIGHT\"},\"type\":\"ConnectorPlacement.EquallySpacedRectSide\",\"uuid\":\"9f78cd75-5645-4950-8d66-9f0d33627f1f\"},{\"content\":{\"connectorIds\":[\"Out6\",\"Out2\",\"Out3\",\"LConn1\",\"Out4\",\"Out5\",\"In5\",\"In2\",\"In3\",\"LConn2\",\"In4\"],\"side\":\"TOP\"},\"type\":\"ConnectorPlacement.EquallySpacedRectSide\",\"uuid\":\"f95077c9-4a6b-4bf1-8b13-59697d659817\"},{\"content\":{\"connectorIds\":[\"RConn1\",\"RConn2\"],\"side\":\"BOTTOM\"},\"type\":\"ConnectorPlacement.EquallySpacedRectSide\",\"uuid\":\"0eafd906-a166-4c55-8e00-9a076c1e2d64\"}]},\"type\":\"ConnectorPlacement.EquallySpacedConnector\",\"uuid\":\"da1ef182-4ed3-4fb4-823f-e8eb0a5ecd15\"}],\"packageUris\":[\"http://schema.mathworks.com/mf0/Connector/R2020b\"],\"version\":\"1.0\"}"
  20X-525FO : PMIOPort  Side=Left  ConnectionType=Bus: FuelOil_P
  525-20XFO : PMIOPort  Port=2  Side=Left  ConnectionType=Bus: FuelOil_P
  TO 23X : PMIOPort  Port=3  Side=Left  ConnectionType=Bus: Physical
  10X-20X : PMIOPort  Port=4  Side=Right  ConnectionType=Bus: Physical
  FROM 20X : PMIOPort  Port=5  Side=Right  ConnectionType=Bus: Physical
  20X-42XC : Outport  OutDataTypeStr=Bus: Control_S
  20X-51XLO : Outport  Port=2  OutDataTypeStr=Bus: LubeOil_S
  20X-52XFO : Outport  Port=3  OutDataTypeStr=Bus: FuelOil_S
  20X-53XCA : Outport  Port=4  OutDataTypeStr=Bus: CompAir_S
  20X-57XWG : Outport  Port=5  OutDataTypeStr=Bus: WasteGas_S
  20X-50XCFW : Outport  Port=6  OutDataTypeStr=Bus: CoolingFW_S
